simulink model "4th_order_plant_test"  (R2021a)
settings: Solver=VariableStepAuto  StartTime=0.0  StopTime=20  MaxStep=0.01  RelTol=1e-13
libraries: adrc_toolbox_library x1, simulink x1
settings Model: Creator=krzys  LastModifiedBy=krzys
settings SolverCC: AlgebraicLoopSolver=TrustRegion
settings DebuggingCC: ArithmeticOperatorsInVariantConditions=warning
settings SFSimCC: CustomCodeUndefinedFunction=UseInterfaceOnly

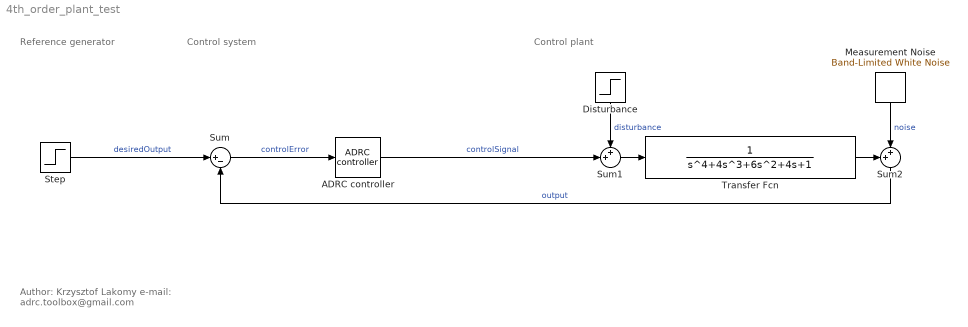
== system 4th_order_plant_test ==
  note: Reference
      | generator
  note: Control system
  note: Control plant
  note: Author: Krzysztof Lakomy
      | e-mail: adrc.toolbox@gmail.com
  ADRC controller : adrc_toolbox_library/ADRC controller  dynamicsOrder=4  controllerBandwidth=5  controllerBandwidthSource=Internal  observerBandwidth=50  observerBandwidthSource=Internal  inputGainParameter=0.8  inputGainSource=Internal  saturationEnabled=on  UpperLimit=100  LowerLimit=-100  deadTimeEnabled=off  deadTime=0.2
      settings: SourceProductName=ADRC Toolbox
  Disturbance : Step  Time=10  After=70  SampleTime=0
  Measurement Noise : simulink/Sources/Band-Limited White Noise  Cov=1e-14  Ts=0.01  seed=[23341]
  Step : Step  SampleTime=0
  Sum : Sum  Inputs=|+-
  Sum1 : Sum  Inputs=++|
  Sum2 : Sum  Inputs=++|
  Transfer Fcn : TransferFcn  Denominator=[1 4 6 4 1]
  wires:
  Sum/1 -> ADRC controller/1  "controlError"
  Transfer Fcn/1 -> Sum2/1
  Sum1/1 -> Transfer Fcn/1
  Disturbance/1 -> Sum1/1  "disturbance"
  ADRC controller/1 -> Sum1/2  "controlSignal"
  Sum2/1 -> Sum/2  "output"
  Measurement Noise/1 -> Sum2/2  "noise"
  Step/1 -> Sum/1  "desiredOutput"
